simulink model "SSLD1"  (Simulink 8.1)
settings: Solver=ode3  StartTime=0.0  StopTime=2  FixedStep=1e-3  RelTol=1e-3
undefined symbols (not defined in the file or in its folder): cutoff_SSLD1
libraries: dspxfrm3 x2, dsparch4 x1
settings Model: Creator=user  LastModifiedBy=Andrew
settings DebuggingCC: FcnCallInpInsideContextMsg=EnableAllAsWarning
settings RTWCC: TargetLang=C++
settings GRTTargetCC: CombineOutputUpdateFcns=on  GRTInterface=off

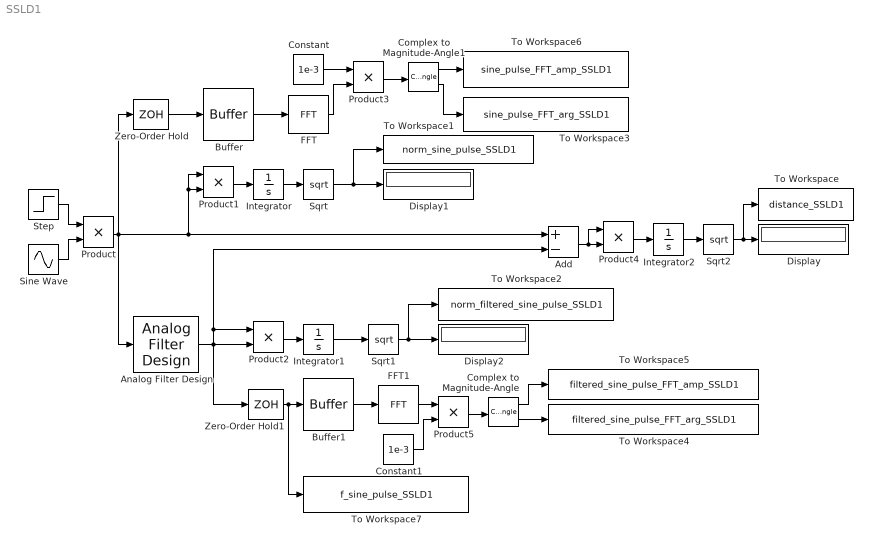
== system SSLD1 ==
  Add : Sum  Inputs=+-
  Analog Filter Design : dsparch4/Analog Filter Design  method=Butterworth  filttype=Lowpass  N=2  Wlo=cutoff_SSLD1*2*pi  Whi=80  Rp=2  Rs=40
  Buffer : Buffer  N=2000  TreatMby1Signals=One channel
  Buffer1 : Buffer  N=2000  TreatMby1Signals=One channel
  Complex to Magnitude-Angle : ComplexToMagnitudeAngle
  Complex to Magnitude-Angle1 : ComplexToMagnitudeAngle
  Constant : Constant  Value=1e-3
  Constant1 : Constant  Value=1e-3
  Display : Display
  Display1 : Display
  Display2 : Display
  FFT : dspxfrm3/FFT  CompMethod=Table lookup  TableOpt=NEW  TableOptActive=Speed  BitRevOrder=off  InheritFFTLength=on  FFTLength=64  RowConvenienceOn=on  FFTImplementation=FFTW  SkipNorm=off  firstCoeffDataTypeStr=Inherit: Same word length as input  firstCoeffLastDataTypeStr=Inherit: Same word length as input  outputMin=[]  outputMax=[]  roundingMode=Floor  overflowMode=off
  FFT1 : dspxfrm3/FFT  CompMethod=Table lookup  TableOpt=NEW  TableOptActive=Speed  BitRevOrder=off  InheritFFTLength=on  FFTLength=64  RowConvenienceOn=on  FFTImplementation=FFTW  SkipNorm=off  firstCoeffDataTypeStr=Inherit: Same word length as input  firstCoeffLastDataTypeStr=Inherit: Same word length as input  outputMin=[]  outputMax=[]  roundingMode=Floor  overflowMode=off
  Integrator : Integrator
  Integrator1 : Integrator
  Integrator2 : Integrator
  Product{,1..5} (6 alike) : Product  RndMeth=Zero
  Sine Wave : Sin  Frequency=2*pi*10  SampleTime=0
  Sqrt : Sqrt  SaturateOnIntegerOverflow=on
  Sqrt1 : Sqrt  SaturateOnIntegerOverflow=on
  Sqrt2 : Sqrt  SaturateOnIntegerOverflow=on
  Step : Step  Time=0.05  Before=1  After=0  SampleTime=0
  To Workspace : ToWorkspace  VariableName=distance_SSLD1  SampleTime=-1
      settings: MaxDataPoints=1
  To Workspace1 : ToWorkspace  VariableName=norm_sine_pulse_SSLD1  SampleTime=-1
      settings: MaxDataPoints=1
  To Workspace2 : ToWorkspace  VariableName=norm_filtered_sine_pulse_SSLD1  SampleTime=-1
      settings: MaxDataPoints=1
  To Workspace3 : ToWorkspace  VariableName=sine_pulse_FFT_arg_SSLD1  SampleTime=-1
      settings: MaxDataPoints=200000
  To Workspace4 : ToWorkspace  VariableName=filtered_sine_pulse_FFT_arg_SSLD1  SampleTime=-1
      settings: MaxDataPoints=200000
  To Workspace5 : ToWorkspace  VariableName=filtered_sine_pulse_FFT_amp_SSLD1  SampleTime=-1
      settings: MaxDataPoints=200000
  To Workspace6 : ToWorkspace  VariableName=sine_pulse_FFT_amp_SSLD1  SampleTime=-1
      settings: MaxDataPoints=2000000
  To Workspace7 : ToWorkspace  VariableName=f_sine_pulse_SSLD1  SampleTime=-1
      settings: MaxDataPoints=2000000
  Zero-Order Hold : ZeroOrderHold  SampleTime=1e-3
  Zero-Order Hold1 : ZeroOrderHold  SampleTime=1e-3
  wires:
  Sine Wave/1 -> Product/2
  Step/1 -> Product/1
  Product1/1 -> Integrator/1
  Integrator/1 -> Sqrt/1
  Product2/1 -> Integrator1/1
  Integrator1/1 -> Sqrt1/1
  Add/1 -> Product4/1, Product4/2
  Integrator2/1 -> Sqrt2/1
  Sqrt2/1 -> Display/1, To Workspace/1
  Analog Filter Design/1 -> Product2/2, Product2/1, Add/2, Zero-Order Hold1/1
  Product4/1 -> Integrator2/1
  Sqrt/1 -> Display1/1, To Workspace1/1
  Sqrt1/1 -> Display2/1, To Workspace2/1
  Product/1 -> Analog Filter Design/1, Zero-Order Hold/1, Product1/1, Product1/2, Add/1
  Buffer/1 -> FFT/1
  Zero-Order Hold/1 -> Buffer/1
  FFT/1 -> Product3/2
  Buffer1/1 -> FFT1/1
  FFT1/1 -> Product5/1
  Zero-Order Hold1/1 -> To Workspace7/1, Buffer1/1
  Constant/1 -> Product3/1
  Constant1/1 -> Product5/2
  Product5/1 -> Complex to Magnitude-Angle/1
  Complex to Magnitude-Angle/2 -> To Workspace4/1
  Complex to Magnitude-Angle/1 -> To Workspace5/1
  Product3/1 -> Complex to Magnitude-Angle1/1
  Complex to Magnitude-Angle1/1 -> To Workspace6/1
  Complex to Magnitude-Angle1/2 -> To Workspace3/1
